simulink library "discretizing"  (Simulink 5.0)
PostLoadFcn:
  | sldiscutil('hide_TransportDelay',gcs)
values from neighbouring files (symbols this model uses):
  A = tmpargin{4}    [sldiscutil.m]
  Ad = get(discsys,'A')    [sldiscutil.m]
  B = tmpargin{5}    [sldiscutil.m]
  Bd = get(discsys,'B')    [sldiscutil.m]
  C = tmpargin{6}    [sldiscutil.m]
  Cd = get(discsys,'C')    [sldiscutil.m]
  D = tmpargin{7}    [sldiscutil.m]
  Dd = get(discsys,'D')    [sldiscutil.m]
  dend = dendc{1}    [sldiscutil.m]
  gaind = get(md,'k')'    [sldiscutil.m]
  icd = G*xarg    [sldiscutil.m]
  numd = numdc{1}    [sldiscutil.m]
  polesd = polesdc{1}'    [sldiscutil.m]
  zerosd = zerosdc{1}'    [sldiscutil.m]
undefined symbols (not defined in the file or in its folder): magnitude, Ts, X0
libraries: cstextras x2, simulink x1, dspbdsp2 x1
settings Model: ProdHWCharacteristics=Microprocessor  Creator=lqin  LastModifiedBy=jwu
settings Model: ForwardingTableString=|
  | ||__slOldName__||discretizing/Discretized
  | Transport Delay 2||__slNewName__||discretizing/Discretized
  | Transport Delay

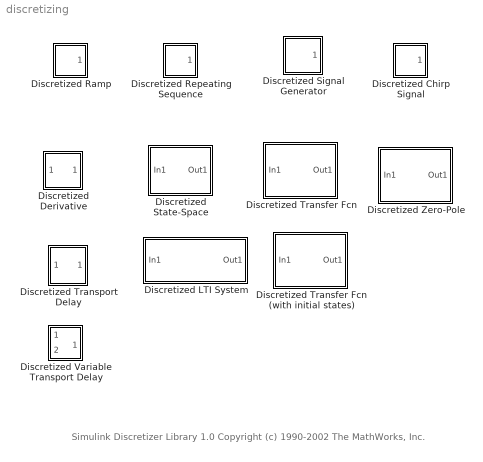
== system discretizing ==
  note: Simulink Discretizer Library 1.0
      | Copyright (c) 1990-2002 The MathWorks, Inc.
  Discretized Chirp Signal : Subsystem  mask(discretizedchirp){f1=0.1, T=50, f2=20, VectorParams1D=on, SampleTime=1}
      mask prompts: f1 "Initial frequency (Hz):"; T "Target time (secs):"; f2 "Frequency at target time (Hz):"; VectorParams1D "Interpret vectors parameters as 1-D"; SampleTime "Sample Time"
      mask help: Output a linear chirp signal (sine wave whose frequency varies linearly with time).
      mask init:
      | t=[0:.1:5];
      | set_param([gcb '/startTime'], 'VectorParams1D', VectorParams1D);
      | set_param([gcb '/targetTime'], 'VectorParams1D', VectorParams1D);
      | set_param([gcb '/initialFreq'], 'VectorParams1D', VectorParams1D);
      | set_param([gcb '/deltaFreq'], 'VectorParams1D', VectorParams1D);
      | st=SampleTime;
      | if length(st)>1
      |     st=SampleTime(1);
      | end
      | sldiscutil('initchirpmask', st);
      mask Help: The chirp signal has linearly increasing frequency with time.  This block can be used for spectral analysis of nonlinear systems.
      mask Display: plot(t,sin(t.*t))
  Discretized Derivative : Subsystem  mask(DiscretizedDerivative){method=tustin, SampleTime=1, Wc=1}
      mask prompts: SampleTime "Sample time:"; Wc "Critical Frequency (Hz):"
      mask help: Continuous mask uses c2d to transform an 's' transfer function onto a Discrete Transfer function block inside at the sample time specified.
      mask init:
      | st=SampleTime;
      | if length(st)>1
      |     st=SampleTime(1);
      | end
      | Numerator = [1 0];
      | Denominator = [1];
      | if(st>0)
      | %	if(strcmpi(method, 'zoh') | strcmpi(method, 'foh'))
      | %       [numd, dend] = sldiscutil('disctransferfcn', {st, 'tustin', Wc, Numerator, Denominator});
      | %	else
      |     [numd, dend] = sldiscutil('disctransferfcn', {st, method, Wc, Numerator, Denominator});
      | %	end
      | end
      | s = get_param(gcb,'maskvalues');
      | nums = s{1};
      | dens = s{2};
      | sldiscutil('initderivativemask', st);
      mask StyleString: popup(zoh|foh|tustin|prewarp|matched),edit,edit
      mask CallbackString: hidecrit||
      mask Display:
      | text( 0.5, 0.45, 'du/dt', 'horizontalAlignment','center')
      | text( 0.5, 1.0, method,'verticalAlignment','top')
  Discretized LTI System : Subsystem  mask(DiscretizedLTISystem){sysc=ss(tf(1,[1 1])), cic=0, SampleTime=1, method=tustin, Wc=0}
      mask prompts: sysc "System (enter in s-domain):"; cic "Initial conditions (enter in s-domain):"; SampleTime "Sample time (enter in s-domain):"; method "Method (enter in s-domain):"; Wc "Critical frquency(Hz) (enter in s-domain):"
      mask help: Continuous mask uses c2d to transform parameters onto the Discrete block parameters.
      mask init:
      | st=SampleTime;
      | 
      | 
      | 
      | 
      | 
      | 
      | 
      | if length(st)>1
      | 
      | 
      | 
      | 
      | 
      | 
      | 
      |     st=SampleTime(1);
      | 
      | 
      | 
      | 
      | 
      | 
      | 
      | end
      | 
      | 
      | 
      | 
      | 
      | 
      | 
      | if(isa(sysc,'ss'))
      | 
      | 
      | 
      | 
      | 
      | 
      | 
      |     set_param(gcb, 'MaskEnables',{'on','on','on','on','on'});
      | 
      | 
      | 
      | 
      | 
      | 
      | 
      | else
      | 
      | 
      | 
      | 
      | 
      | 
      | 
      | 	set_param(gcb, 'MaskEnables',{'on','off','on','on','on'});
      | 
      | 
      | 
      | 
      | 
      | 
      | 
      | end
      | 
      | 
      | 
      | 
      | 
      | 
      | 
      | 
      | 
      | 
      | 
      | 
      | 
      | 
      | 
      | if st > 0
      | 
      | 
      | 
      | 
      | 
      | 
      | 
      | 	[discsys, discic] = sldiscutil('disclti', {st, method, Wc, sysc, cic});
      | 
      | 
      | 
      | 
      | 
      | 
      | 
      | else
      | 
      | 
      | 
      | 
      | 
      | 
      | 
      | 	discsys = sysc;
      | 
      | 
      | 
      | 
      | 
      | 
      | 
      | 	discic = 0;
      | 
      | 
      | 
      | 
      | 
      | 
      | 
      | end
      | 
      | 
      | 
      | 
      | 
      | 
      | 
      | 
      | 
      | 
      | 
      | 
      | 
      | 
      | 
      | ltiblk = sprintf('%s/LTI System',gcb);
      | 
      | 
      | 
      | 
      | 
      | 
      | 
      | try
      | 
      | 
      | 
      | 
      | 
      | 
      | 
      | % set_param(ltiblk, 'sys', 'discsys');
      | 
      | 
      | 
      | 
      | 
      | 
      | 
      | set_param(ltiblk, 'IC', 'discic');
      | 
      | 
      | 
      | 
      | 
      | 
      | 
      | catch
      | 
      | 
      | 
      | 
      | 
      | 
      | 
      | end
      mask StyleString: edit,edit,edit,popup(zoh|foh|tustin|prewarp|matched|imp),edit
      mask CallbackString: |||hidecrit|
      mask Display:
      | disp(get_param(gcb, 'sysc'))
      | 
      | 
      | 
      | 
      | 
      | 
      | 
      | text( 0.5, 1.0, method, 'verticalAlignment','top')
  Discretized Ramp : Subsystem  mask(DiscretizedRamp){slope=1, start=0, X0=0, SampleTime=1}
      mask prompts: start "Start time:"; X0 "Initial output:"; SampleTime "Sample time:"
      mask help: ramp
      mask init:
      | curblkc  = find_system(gcb,'FollowLinks','on','LookUnderMasks','all','searchdepth', 1, 'BlockType','Clock');
      | 
      | 
      | 
      | 
      | 
      | 
      | 
      | curblkdc = find_system(gcb,'FollowLinks','on','LookUnderMasks','all','searchdepth', 1, 'BlockType','DigitalClock');
      | 
      | 
      | 
      | 
      | 
      | 
      | 
      | st=SampleTime;
      | 
      | 
      | 
      | 
      | 
      | 
      | 
      | if length(st)>1
      | 
      | 
      | 
      | 
      | 
      | 
      | 
      |     st=SampleTime(1);
      | 
      | 
      | 
      | 
      | 
      | 
      | 
      | end
      | 
      | 
      | 
      | 
      | 
      | 
      | 
      | sldiscutil('initrampmask', st);
      mask Display: plot([0:10],[1,1,1,1:8])
  Discretized Repeating Sequence : Subsystem  mask(DiscretizedRepeatingTable){rep_seq_t=[0 2], rep_seq_y=[0 2], SampleTime=1}
      mask prompts: rep_seq_t "Time values:"; rep_seq_y "Output values:"; SampleTime "Sample time:"
      mask help: Repeating table.
      mask init:
      | period = max(rep_seq_t);
      | st=SampleTime;
      | if length(st)>1
      |     st=SampleTime(1);
      | end
      | sldiscutil('initrepeatsequencemask', st);
      mask Help: Repeats cycle given in table. Time values should be monotonically increasing.
      mask Display: plot([rep_seq_t,rep_seq_t+period,rep_seq_t+2*period,rep_seq_t(1)+3*period],[rep_seq_y,rep_seq_y,rep_seq_y,rep_seq_y(1)])
  Discretized Signal Generator : Subsystem  mask(DiscretizedSignalGenerator){WaveForm=sine, Amplitude=1, Frequency=1, Units=Hertz, SampleTime=0.1}
      mask prompts: SampleTime "Sample time:"
      mask help: A discrete equivalent to the Signal Generator Block.
      mask init:
      | xdrw = 11*[1,1,2,2,1];
      | ydrw = [72,88,88,72,72];
      | xcirc = 11*[0,0,0.25,0.75,1,1,0.75,0.25,0];
      | ycirc = 16*[0.25,0.75,1,1,0.75,0.25,0,0,0.25];
      | switch Units
      |   case 'rad/sec'
      |     frequencyHz = Frequency/(2*pi);
      |     frequencyRads = Frequency;
      |   case 'Hertz'
      |     frequencyHz = Frequency;
      |     frequencyRads = Frequency*2*pi;
      | end
      | Period = 1.0/frequencyHz;
      | st=SampleTime;
      | DupSampleTime = SampleTime;
      | if length(SampleTime) > 1
      |     st=SampleTime(1);
      | end
      | %discretePeriod = round(period/st);
      | %pulseWidth = round(period*duty/100/st);
      | %phaseDelay =round(start/st);
      | %SampleTime=st;
      | if(st > 0)
      |     PeriodSamples = max(2,round(Period/st));
      |     halfSamples = max(1,round(PeriodSamples/2));
      | else
      | 	PeriodSamples = 2;
      |     halfSamples = 1;
      | end
      | 
      | sldiscutil('initsiggenmask', st);
      mask StyleString: popup(sine|square|sawtooth|random),edit,edit,popup(rad/sec|Hertz),edit
      mask Display:
      | plot( 1,1,99,99,   0+xdrw, ydrw );
      | plot( 1,1,99,99, 22+xdrw, ydrw );
      | plot( 1,1,99,99, 44+xdrw, ydrw );
      | plot( 1,1,99,99, 66+xdrw, ydrw );
      | plot( 1,1,99,99, 22+xcirc, 44+ycirc );
      | plot( 1,1,99,99, 44+xcirc, 44+ycirc );
  Discretized State-Space : Subsystem  mask(DiscretizedStateSpace){A=1, B=1, C=1, D=1, ic=0, AbsTol=auto, SampleTime=1, method=tustin, Wc=1}
      mask prompts: A "A (enter in s-domain:)"; B "B (enter in s-domain:)"; C "C (enter in s-domain:)"; D "D (enter in s-domain:)"; ic "Initial conditions (enter in s-domain:)"; AbsTol "Absolute tolerance"; SampleTime "Sample time:"; Wc "Critical Frequency (Hz):"
      mask help: Continuous mask uses c2d to transform parameters onto the Discrete State-Space block inside.
      mask init:
      | st=SampleTime;
      | if length(st)>1
      |     st=SampleTime(1);
      | end
      | if(st>0)
      |     [Ad, Bd, Cd, Dd, icd] = sldiscutil('discstatespace', {st,method,Wc,A,B,C,D,ic});
      | end
      | sldiscutil('initssmask', st);
      | if(st==0)
      | set_param([gcb '/State Space'], 'AbsoluteTolerance', AbsTol);
      | end
      mask StyleString: edit,edit,edit,edit,edit,edit,edit,popup(zoh|foh|tustin|prewarp|matched),edit
      mask CallbackString: |||||||hidecrit|
      mask Display:
      | text( 0.5, 0.65, 'x'' = Ax+Bu', 'horizontalAlignment', 'center');
      | text( 0.5, 0.4, 'y = Cx+Du', 'horizontalAlignment', 'center');
      | text( 0.5, 1.0, method, 'verticalAlignment', 'top')
  Discretized Transfer Fcn : Subsystem  mask(DiscretizedTransferFcn){Numerator=[1], Denominator=[1 1], AbsTol=auto, SampleTime=1, method=tustin, Wc=1}
      mask prompts: Numerator "Numerator (enter in s-domain:)"; Denominator "Denominator (enter in s-domain:)"; AbsTol "Absolute tolerance:"; SampleTime "Sample time:"; Wc "Critical Frequency (Hz):"
      mask help: Continuous mask uses c2d to transform parameters onto the Discrete Transfer function block inside.
      mask init:
      | st=SampleTime;
      | if length(st)>1
      |     st=SampleTime(1);
      | end
      | if(st>0)
      |     [numd,dend] = sldiscutil('disctransferfcn',{st,method,Wc,Numerator,Denominator});
      | end	
      | s = get_param(gcb,'maskvalues');
      | nums = s{1};
      | dens = s{2};
      | %numc = eval(nums);
      | %denc = eval(dens);
      | sldiscutil('inittfmask', st);
      | if(st==0)
      | set_param([gcb '/Transfer Fcn'], 'AbsoluteTolerance', AbsTol);
      | end
      mask StyleString: edit,edit,edit,edit,popup(zoh|foh|tustin|prewarp|matched),edit
      mask CallbackString: ||||hidecrit|
      mask Display:
      | dpoly(nums,dens)
      | text( 0.5, 1.0, method, 'verticalAlignment','top')
  Discretized Transfer Fcn (with initial states) : Subsystem  mask(DiscretizedTransferFcnWithIC){Numerator=[1], Denominator=[1 1], X0=auto, SampleTime=1, method=tustin, Wc=1}
      mask prompts: Numerator "Numerator (enter in s-domain:)"; Denominator "Denominator (enter in s-domain:)"; X0 "Initial conditions:"; SampleTime "Sample time:"; Wc "Critical Frequency (Hz):"
      mask help: Continuous mask uses c2d to transform parameters onto the Discrete Transfer function block inside.
      mask init:
      | st=SampleTime;
      | if length(st)>1
      |     st=SampleTime(1);
      | end
      | if(st>0)
      |     [numd,dend] = sldiscutil('disctransferfcn',{st,method,Wc,Numerator,Denominator});
      | end	
      | s = get_param(gcb,'maskvalues');
      | nums = s{1};
      | dens = s{2};
      | %numc = eval(nums);
      | %denc = eval(dens);
      | sldiscutil('inittfmask', st);
      | %if(st==0)
      | %set_param([gcb '/Transfer Fcn'], 'X0', X0);
      | %end
      mask StyleString: edit,edit,edit,edit,popup(zoh|foh|tustin|prewarp|matched),edit
      mask CallbackString: ||||hidecrit|
      mask Display:
      | dpoly(nums,dens)
      | text( 0.5, 1.0, method, 'verticalAlignment','top')
  Discretized Transport Delay : Subsystem  mask(DiscretizedTransportDelay){delay=1, ic=0, SampleTime=1, rounding=Floor}
      mask prompts: delay "Delay (sec):"; ic "Initial value:"; SampleTime "Sample time:"; rounding "Round toward:"
      mask help: Uses either an integer delay or a Discrete State Space Transfer Function for fractional delays internally to mimic the behavior of a continuous transport delay.
      mask init:
      | n = 10;t = 0:pi/n:2.25*pi;pshift = floor(2*n/3);
      | st=SampleTime;
      | if length(st)>1
      |    st=SampleTime(1);
      | end
      | if(st>0)
      |  	if (abs(delay/st-round(delay/st)) < eps*abs(delay/st)) | rounding == 3
      | 		samples=round(delay/st);
      | 	elseif rounding == 1
      | 		samples = floor(delay/st);
      | 	elseif rounding == 2
      | 		samples = ceil(delay/st);
      | 	else
      | 		samples=delay/st;
      | 		if (rounding == 5)
      | 			samples = samples - 1;
      | 		end
      | 		N = floor(samples)+1;
      | 		den = 1;
      | 		num = 1;
      | 		ct = 0:N;
      | 		for k = 1:N
      | 			ak = ((-1)^k)*factorial(N)/(factorial(k)*factorial(N-k))...
      | 				*prod((samples-N+ct)./(samples-N+k+ct));
      | 			num = [ak num];
      | 			den = [den ak];
      | 		end
      | 		if (rounding == 5)
      | 			den = [den 0];
      | 			samples=delay/st;
      | if samples<1
      | samples = 1;
      | end
      | 		end
      | 		[A,B,C,Dd] = tf2ss(num,den);
      | 		if (isempty(ic))
      | 			ic = zeros(1,size(A,1));
      | 		end
      | 	end
      | else
      | 	samples = 0;
      | end
      | sldiscutil('inittransdelaymask', samples);
      settings: AttributesFormatString=(Round to %<rounding>)
      mask Help: An Integer Delay block is used whenever rounding is performed (Floor, Ceiling, or Nearest), or when the Delay divided by the Sample time is an integer.  If the Fractional Delay is chosen, a Discrete State Space Transfer Function is developed using the Thiran filter algorithm to approximate the continuous Transport Delay.  When the Fractional Delay (no Dir. FT) option is selected, the Thiran filter is approximated to accomodate systems requiring no direct feedthrough (such as algebraic loops).  If the Delay is less than the Sample time, then an Integer Delay of one is used.
      mask StyleString: edit,edit,edit,popup(Floor|Ceiling|Nearest|Fractional Delay|Fractional Delay (no direct FT))
      mask Display:
      | plot(t, sin(t))
      | plot(t(pshift+1:end),sin(t(1:end-pshift)))
      | plot([0 t(pshift+1)],[0 0])
      | plot([3 4.2 4 4 4.2],[.4 .4 .46 .34 .4])
      | plot([3.9 5.1 4.9 4.9 5.1],-[.4 .4 .46 .34 .4])
  Discretized Variable Transport Delay : Subsystem  mask(DiscretizedVarTransDelay){MaximumDelay=1, InitialInput=0, MaximumPoints=1024, SampleTime=1}
      mask prompts: MaximumDelay "Maximum delay (sec):"; InitialInput "Initial input:"; MaximumPoints "Buffer size:"; SampleTime "Sample time:"
      mask help: Uses a Z^-k variable delay line to mimic the behavior of the continuous variable transport delay block.
      mask init:
      | st=SampleTime;
      | if length(st)>1
      |      st=SampleTime(1);
      | end
      | if(st>0)
      |     maxDelaySamples=ceil(MaximumDelay/st);
      | else
      | 	maxDelaySamples = 0;
      | end
      | pos = get_param(gcb,'Position');
      | width = pos(3) - pos(1);
      | height = pos(4) - pos(2);
      | expWidth = 2;
      | sldiscutil('initvartransdelaymask', st);
      mask Help: Note: the Buffer size parameter is included only for holding the parameter value in case of conversion back to the continuous variable transport delay.
      mask Display:
      | text(width/2-3*expWidth, height/2, 'z');
      | text(width/2-3*(expWidth-1), height/2+5, '-k');
  Discretized Zero-Pole : Subsystem  mask(DiscretizedZeroPole){Zeros=[1], Poles=[1 1], Gain=[2], AbsTol=auto, SampleTime=1, method=tustin, Wc=1}
      mask prompts: Zeros "Zeros (enter in s-main:)"; Poles "Poles (enter in s-domain:)"; Gain "Gain (enter in s-domain:)"; AbsTol "Absolute tolerance:"; SampleTime "Sample time:"; Wc "Critical Frequency (Hz):"
      mask help: Continuous mask uses c2d to transform parameters onto the Discrete Zero-Pole block inside.
      mask init:
      | st=SampleTime;
      | if length(st)>1
      |     st=SampleTime(1);
      | end
      | if(st>0)
      |     [zerosd,polesd,gaind] = sldiscutil('disczpk', {st,method,Wc,Zeros,Poles,Gain});
      | end	
      | s = get_param(gcb,'maskvalues');
      | zeross = s{1};
      | poless = s{2};
      | gainss = s{3};
      | %zerosc = eval(zeross);
      | %polesc = eval(poless);
      | %gainsc = eval(gainss);
      | sldiscutil('initzpkmask', st);
      | if(st==0)
      | set_param([gcb '/Zero Pole'], 'AbsoluteTolerance', AbsTol);
      | end
      mask StyleString: edit,edit,edit,edit,edit,popup(zoh|foh|tustin|prewarp|matched),edit
      mask CallbackString: |||||hidecrit|
      mask Display:
      | droots(zeross,poless,gainss)
      | text( 0.5, 1.0, method, 'verticalAlignment','top')

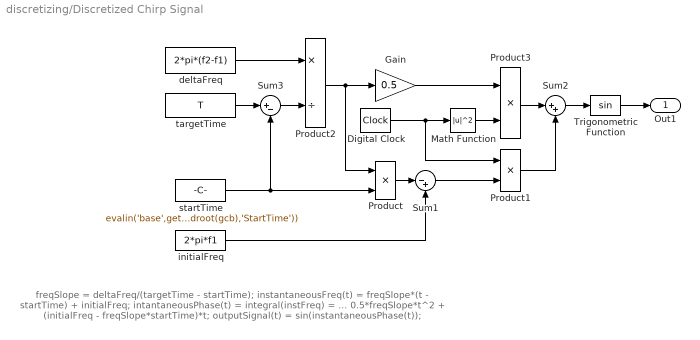
== system discretizing/Discretized Chirp Signal ==
  note: freqSlope = deltaFreq/(targetTime - startTime);
      | instantaneousFreq(t) = freqSlope*(t - startTime) + initialFreq;
      | intantaneousPhase(t) = integral(instFreq) = ...
      |       0.5*freqSlope*t^2 + (initialFreq - freqSlope*startTime)*t;
      | outputSignal(t) = sin(instantaneousPhase(t));
  Digital Clock : DigitalClock  SampleTime=SampleTime
  Gain : Gain  Gain=0.5  SaturateOnIntegerOverflow=on
  Math Function : Math  Operator=magnitude^2
  Product : Product  SaturateOnIntegerOverflow=on  InputSameDT=on
  Product1 : Product  SaturateOnIntegerOverflow=on  InputSameDT=on
  Product2 : Product  Inputs=*/  SaturateOnIntegerOverflow=on  InputSameDT=on
  Product3 : Product  SaturateOnIntegerOverflow=on  InputSameDT=on
  Sum1 : Sum  Inputs=|-+  SaturateOnIntegerOverflow=on  InputSameDT=on
  Sum2 : Sum  Inputs=|++  SaturateOnIntegerOverflow=on  InputSameDT=on
  Sum3 : Sum  Inputs=|+-  SaturateOnIntegerOverflow=on  InputSameDT=on
  Trigonometric Function : Trigonometry
  deltaFreq : Constant  Value=2*pi*(f2-f1)
  initialFreq : Constant  Value=2*pi*f1
  startTime : Constant  Value=evalin('base',get_param(bdroot(gcb),'StartTime'))
  targetTime : Constant  Value=T
  Out1 : Outport
  wires:
  Digital Clock/1 -> Product1/1, Math Function/1
  Product2/1 -> Gain/1, Product/1
  deltaFreq/1 -> Product2/1
  Sum3/1 -> Product2/2
  targetTime/1 -> Sum3/1
  startTime/1 -> Sum3/2, Product/2
  Trigonometric Function/1 -> Out1/1
  Product/1 -> Sum1/1
  Sum2/1 -> Trigonometric Function/1
  Product3/1 -> Sum2/1
  Product1/1 -> Sum2/2
  Sum1/1 -> Product1/2
  Gain/1 -> Product3/1
  Math Function/1 -> Product3/2
  initialFreq/1 -> Sum1/2

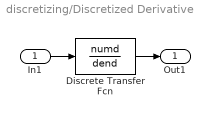
== system discretizing/Discretized Derivative ==
  In1 : Inport
  Discrete Transfer Fcn : DiscreteTransferFcn  Numerator=numd  Denominator=dend  SampleTime=SampleTime
  Out1 : Outport
  wires:
  In1/1 -> Discrete Transfer Fcn/1
  Discrete Transfer Fcn/1 -> Out1/1

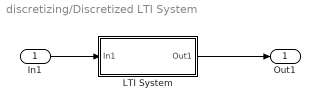
== system discretizing/Discretized LTI System ==
  In1 : Inport
  LTI System : Subsystem  AncestorBlock=cstblocks/LTI System  mask(LTI Block){sys=discsys, IC=discic}
      mask prompts: sys "LTI system variable"; IC "Initial states   (state-space only)"
      mask help:
      | The LTI System block accepts both continuous and discrete LTI models as defined in the Control System Toolbox. Transfer function, state-space, and zero-pole-gain formats are all supported in this block.
      |
      | Note: Initial states are only meaningful for state-space systems.
      mask init:
      | [A,B,C,D,Ts,Tdi,Tdo,X0,sysname]=ltimask('Initialize',gcb,sys,IC);
      mask Help:
      | The LTI System block accepts any of the three standard LTI models described in the Control System Toolbox: transfer function, zero/pole/gain, or state space. Internally, LTI models will be converted to their state space equivalent for evaluation.
      | <p>
      | In the editable text box labeled <b>LTI System Variable</b>, enter a valid LTI model.
      | <p>
      | In the editable text box labeled <b>Initial States</b> enter the initial state vector.  Initial states are only valid for state-space systems.
      | <p>
      | See also TF, ZPK, SS, LTIMODELS.
      mask CallbackString: ltimask('MaskLTICallback',gcb);|
      mask Display: disp(sysname)
  Out1 : Outport
  wires:
  LTI System/1(Out1) -> Out1/1
  In1/1 -> LTI System/1(In1)

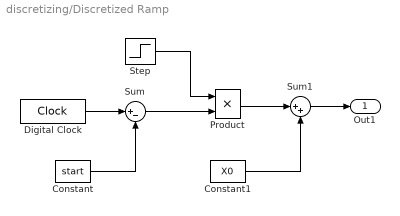
== system discretizing/Discretized Ramp ==
  Constant : Constant  Value=start
  Constant1 : Constant  Value=X0
  Digital Clock : DigitalClock  SampleTime=SampleTime
  Product : Product  SaturateOnIntegerOverflow=on  InputSameDT=on
  Step : Step  Time=start  After=slope  SampleTime=SampleTime
  Sum : Sum  Inputs=|+-  SaturateOnIntegerOverflow=on  InputSameDT=on
  Sum1 : Sum  Inputs=|++  SaturateOnIntegerOverflow=on  InputSameDT=on
  Out1 : Outport
  wires:
  Digital Clock/1 -> Sum/1
  Constant/1 -> Sum/2
  Sum/1 -> Product/2
  Sum1/1 -> Out1/1
  Constant1/1 -> Sum1/2
  Product/1 -> Sum1/1
  Step/1 -> Product/1

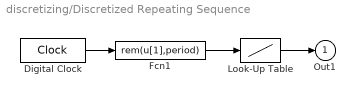
== system discretizing/Discretized Repeating Sequence ==
  Digital Clock : DigitalClock  SampleTime=SampleTime
  Fcn1 : Fcn  Expr=rem(u[1],period)
  Look-Up Table : Lookup  InputValues=rep_seq_t  OutputValues=rep_seq_y  SaturateOnIntegerOverflow=on
  Out1 : Outport
  wires:
  Look-Up Table/1 -> Out1/1
  Digital Clock/1 -> Fcn1/1
  Fcn1/1 -> Look-Up Table/1

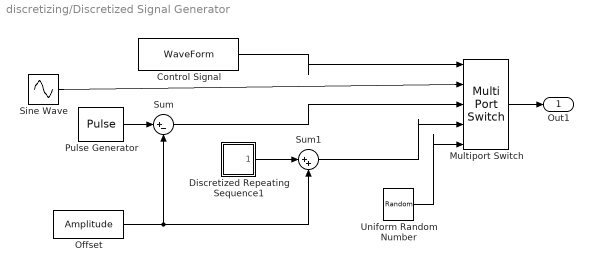
== system discretizing/Discretized Signal Generator ==
  Control Signal : Constant  Value=WaveForm
  Discretized Repeating Sequence1 : Subsystem  AncestorBlock=discretizing/Discretized Repeating Sequence  mask(DiscretizedRepeatingTable){rep_seq_t=[0 Period], rep_seq_y=[0 ((-2)*Amplitude)], SampleTime=DupSampleTime}
      mask prompts: rep_seq_t "Time values:"; rep_seq_y "Output values:"; SampleTime "Sample time:"
      mask help: Repeating table.
      mask init:
      | period = max(rep_seq_t);
      | st=SampleTime;
      | if length(st)>1
      |     st=SampleTime(1);
      | end
      | sldiscutil('initrepeatsequencemask', st);
      mask Help: Repeats cycle given in table. Time values should be monotonically increasing.
      mask Display: plot([rep_seq_t,rep_seq_t+period,rep_seq_t+2*period,rep_seq_t(1)+3*period],[rep_seq_y,rep_seq_y,rep_seq_y,rep_seq_y(1)])
  Multiport Switch : MultiPortSwitch  InputSameDT=on
  Offset : Constant  Value=Amplitude
  Pulse Generator : DiscretePulseGenerator  Amplitude=2*Amplitude  Period=PeriodSamples  PulseWidth=halfSamples  PhaseDelay=halfSamples  SampleTime=st
  Sine Wave : Sin  Amplitude=Amplitude  Frequency=frequencyRads  SampleTime=SampleTime
  Sum : Sum  Inputs=|+-  SaturateOnIntegerOverflow=on  InputSameDT=on
  Sum1 : Sum  Inputs=|++  SaturateOnIntegerOverflow=on  InputSameDT=on
  Uniform Random Number : UniformRandomNumber  Minimum=(-1)*Amplitude  Maximum=Amplitude  SampleTime=SampleTime
  Out1 : Outport
  wires:
  Uniform Random Number/1 -> Multiport Switch/5
  Sine Wave/1 -> Multiport Switch/2
  Control Signal/1 -> Multiport Switch/1
  Pulse Generator/1 -> Sum/1
  Sum/1 -> Multiport Switch/3
  Multiport Switch/1 -> Out1/1
  Discretized Repeating Sequence1/1(Out1) -> Sum1/1
  Sum1/1 -> Multiport Switch/4
  Offset/1 -> Sum1/2, Sum/2

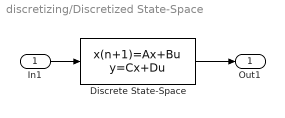
== system discretizing/Discretized State-Space ==
  In1 : Inport
  Discrete State-Space : DiscreteStateSpace  A=Ad  B=Bd  C=Cd  D=Dd  X0=icd  SampleTime=SampleTime
  Out1 : Outport
  wires:
  In1/1 -> Discrete State-Space/1
  Discrete State-Space/1 -> Out1/1

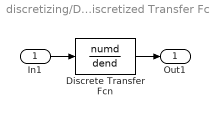
== system discretizing/Discretized Transfer Fcn ==
  In1 : Inport
  Discrete Transfer Fcn : DiscreteTransferFcn  Numerator=numd  Denominator=dend  SampleTime=SampleTime
  Out1 : Outport
  wires:
  Discrete Transfer Fcn/1 -> Out1/1
  In1/1 -> Discrete Transfer Fcn/1

== system discretizing/Discretized Transfer Fcn (with initial states) ==
  In1 : Inport
  Discrete Transfer Fcn : DiscreteTransferFcn  Numerator=numd  Denominator=dend  SampleTime=SampleTime
  Out1 : Outport
  wires:
  In1/1 -> Discrete Transfer Fcn/1
  Discrete Transfer Fcn/1 -> Out1/1

== system discretizing/Discretized Transport Delay ==
  In1 : Inport  SampleTime=SampleTime
  Integer Delay : simulink/Discrete/Integer Delay  NumDelays=samples  vinit=ic  samptime=st
  Out1 : Outport
  wires:
  Integer Delay/1 -> Out1/1
  In1/1 -> Integer Delay/1

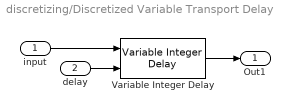
== system discretizing/Discretized Variable Transport Delay ==
  input : Inport  SampleTime=SampleTime
  delay : Inport  Port=2  SampleTime=SampleTime
  Variable Integer Delay : dspbdsp2/Variable Integer Delay  dmax=maxDelaySamples  ic=InitialInput  frame=off  numChans=1
  Out1 : Outport
  wires:
  Variable Integer Delay/1 -> Out1/1
  delay/1 -> Variable Integer Delay/2
  input/1 -> Variable Integer Delay/1

== system discretizing/Discretized Zero-Pole ==
  In1 : Inport
  Discrete Zero-Pole : DiscreteZeroPole  Zeros=zerosd  Poles=polesd  Gain=gaind  SampleTime=SampleTime
  Out1 : Outport
  wires:
  In1/1 -> Discrete Zero-Pole/1
  Discrete Zero-Pole/1 -> Out1/1

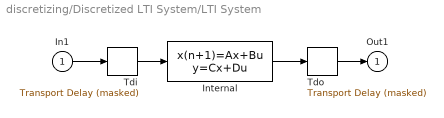
== system discretizing/Discretized LTI System/LTI System ==
  In1 : Inport
  Internal : DiscreteStateSpace  A=A  B=B  C=C  D=D  X0=X0  SampleTime=Ts
  Tdi : cstextras/Transport Delay (masked)  Tag=InputDelayBlock  Td=Tdi  u0=0  bufsize=1024
  Tdo : cstextras/Transport Delay (masked)  Tag=OutputDelayBlock  Td=Tdo  u0=0  bufsize=1024
  Out1 : Outport  InitialOutput=0
  wires:
  Tdo/1 -> Out1/1
  Internal/1 -> Tdo/1
  Tdi/1 -> Internal/1
  In1/1 -> Tdi/1

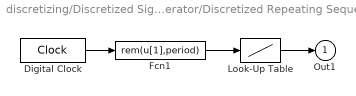
== system discretizing/Discretized Signal Generator/Discretized Repeating Sequence1 ==
  Digital Clock : DigitalClock  SampleTime=SampleTime
  Fcn1 : Fcn  Expr=rem(u[1],period)
  Look-Up Table : Lookup  InputValues=rep_seq_t  OutputValues=rep_seq_y  SaturateOnIntegerOverflow=on
  Out1 : Outport
  wires:
  Fcn1/1 -> Look-Up Table/1
  Digital Clock/1 -> Fcn1/1
  Look-Up Table/1 -> Out1/1
